simulink model "exp5"  (R2024b)
settings: Solver=ode4  StartTime=0.0  StopTime=.1  FixedStep=1e-8  RelTol=1e-3
libraries: spsDiodeLib x8, spsThyristorLib x8, spsSeriesRLCBranchLib x6, spsACVoltageSourceLib x4, spsCurrentMeasurementLib x4, spsMultimeterLib x4, spsMonostableLib x2, simulink x1, sps_lib x1
settings Model: Creator=91798  LastModifiedBy=91798
settings RTWCC: GPUComputeCapability=3.5

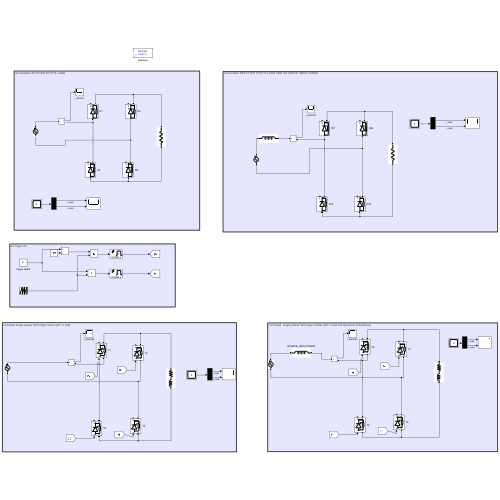
[thumbnail: Simulink's stored preview of the top-level diagram]
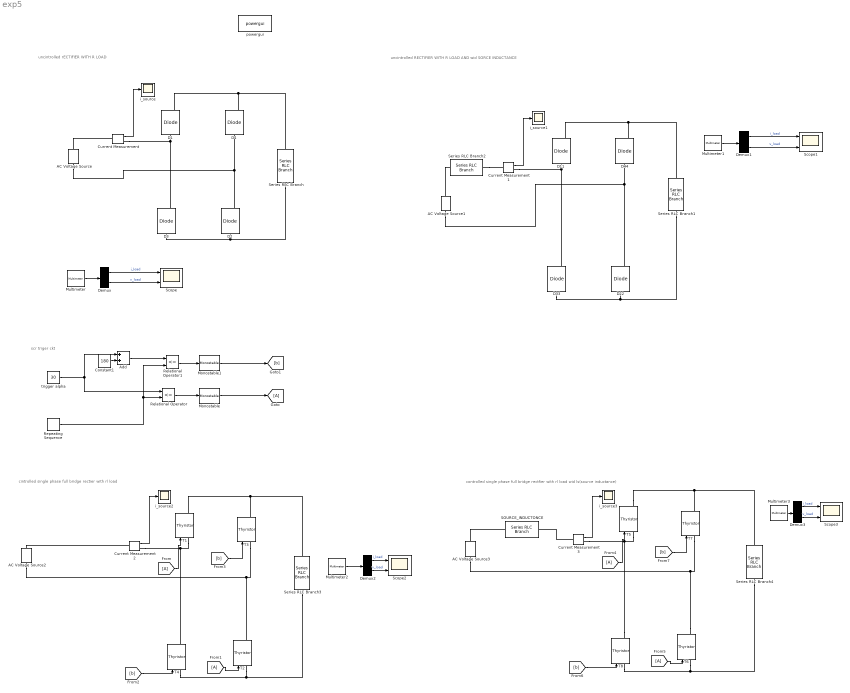
== system exp5 ==
  note: cintrolled single phase full bridge rectier with rl load
  note: controlled single phase full bridge rectfier with rl load wid ls(source inductance)
  note: scr triger ckt
  note: uncintrolled rECTIFIER WITH R LOAD
  note: uncintrolled RECTIFIER WITH R LOAD AND wid SORCE INDUCTANCE
  AC Voltage Source{,1..3} (4 alike) : spsACVoltageSourceLib/AC Voltage Source  Amplitude=230*sqrt(2)  Phase=0  Frequency=50  SampleTime=0  Measurements=None  BusType=swing  Pref=10e3  Qref=0  Qmin=-inf  Qmax=+inf
  Add : Sum
  Constant1 : Constant  Value=180
  Current Measurement{,1..3} (4 alike) : spsCurrentMeasurementLib/Current Measurement  PhasorSimulation=off  OutputType=Complex  PSBequivalent=0
  D{1..4} (4 alike) : spsDiodeLib/Diode  Ron=0.001  Lon=0  Vf=0.8  IC=0  UseSnubber=0  Rs=500  Cs=250e-9  Measurements=on
  D{11,22,33,44} (4 alike) : spsDiodeLib/Diode  Ron=0.001  Lon=0  Vf=0.8  IC=0  UseSnubber=0  Rs=5e10  Cs=inf  Measurements=on
  Demux{,1..3} (4 alike) : Demux  Outputs=2
  From{,1,4..5} (4 alike) : From
  Goto : Goto
  Monostable : spsMonostableLib/Monostable  EdgeDetect=Rising  PulseDuration=0.5e-3  ic=0  Ts=0
      settings: LibrarySourceBlock=sps_lib/Control/Monostable
  Monostable1 : spsMonostableLib/Monostable  EdgeDetect=Rising  PulseDuration=0.5e-3  ic=0  Ts=0
      settings: LibrarySourceBlock=sps_lib/Control/Monostable
  Multimeter : spsMultimeterLib/Multimeter  L=10  sel=[6 1]  yselected={}  Gain=[1 1]  OutputType=Complex  PlotAtSimulationStop=off  PhasorSimulation=off
  Multimeter1 : spsMultimeterLib/Multimeter  L=10  sel=[7 2]  yselected={}  Gain=[1 1]  OutputType=Complex  PlotAtSimulationStop=off  PhasorSimulation=off
  Multimeter2 : spsMultimeterLib/Multimeter  L=10  sel=[9 4]  yselected={}  Gain=[1 1]  OutputType=Complex  PlotAtSimulationStop=off  PhasorSimulation=off
  Multimeter3 : spsMultimeterLib/Multimeter  L=10  sel=[10 5]  yselected={}  Gain=[1 1]  OutputType=Complex  PlotAtSimulationStop=off  PhasorSimulation=off
  Relational Operator : RelationalOperator  Operator=<=  OutDataTypeStr=boolean  InputSameDT=off
  Relational Operator1 : RelationalOperator  Operator=<=  OutDataTypeStr=boolean  InputSameDT=off
  Repeating Sequence : simulink/Sources/Repeating Sequence  rep_seq_t=[0 .02]  rep_seq_y=[0 360]
  SOURCE_INDUCTONCE : spsSeriesRLCBranchLib/Series RLC Branch  LConnTagsString=__new0  RConnTagsString=__new0  BranchType=L  Resistance=20  Inductance=10e-3  SetiL0=off  InitialCurrent=0  Capacitance=1e-6  Setx0=off  InitialVoltage=0  Measurements=None
  Scope{,1..3} (4 alike) : Scope  NumInputPorts=2
  Series RLC Branch : spsSeriesRLCBranchLib/Series RLC Branch  LConnTagsString=__new0  RConnTagsString=__new0  BranchType=R  Resistance=20  Inductance=1e-3  SetiL0=off  InitialCurrent=0  Capacitance=1e-6  Setx0=off  InitialVoltage=0  Measurements=Branch voltage and current
  Series RLC Branch1 : spsSeriesRLCBranchLib/Series RLC Branch  LConnTagsString=__new0  RConnTagsString=__new0  BranchType=R  Resistance=20  Inductance=1e-3  SetiL0=off  InitialCurrent=0  Capacitance=1e-6  Setx0=off  InitialVoltage=0  Measurements=Branch voltage and current
  Series RLC Branch2 : spsSeriesRLCBranchLib/Series RLC Branch  LConnTagsString=__new0  RConnTagsString=__new0  BranchType=L  Resistance=20  Inductance=10e-3  SetiL0=off  InitialCurrent=0  Capacitance=1e-6  Setx0=off  InitialVoltage=0  Measurements=Branch voltage and current
  Series RLC Branch3 : spsSeriesRLCBranchLib/Series RLC Branch  LConnTagsString=__new0  RConnTagsString=__new0  BranchType=RL  Resistance=20  Inductance=200e-3  SetiL0=off  InitialCurrent=0  Capacitance=1e-6  Setx0=off  InitialVoltage=0  Measurements=Branch voltage and current
  Series RLC Branch4 : spsSeriesRLCBranchLib/Series RLC Branch  LConnTagsString=__new0  RConnTagsString=__new0  BranchType=RL  Resistance=20  Inductance=200e-3  SetiL0=off  InitialCurrent=0  Capacitance=1e-6  Setx0=off  InitialVoltage=0  Measurements=Branch voltage and current
  T{1..8} (8 alike) : spsThyristorLib/Thyristor  Ron=0.001  Lon=0  Vf=0.8  IC=0  Rs=500  Cs=250e-9  Measurements=on
  i_source{,1..3} (4 alike) : Scope
  powergui : sps_lib/powergui  Priority=1  SimulationMode=Discrete  SampleTime=5e-7  frequency=60  Iterations=50  frequencyindice=50  Pbase=100e6  ErrMax=1e-4  UnitsV=kV  UnitsW=MW  buscounter=0  FunctionMessages=off  echomessages=off  EnableUseOfTLC=off  CurrentSourceSwitches=off  DisableSnubberDevices=off  DisableRonSwitches=off  DisableVfSwitches=off  DisplayEquations=off  AutomaticDiscreteSolvers=off  SolverType=Tustin/Backward Euler (TBE)  Interpol=off  ExternalGateDelay=off  methode=off  Ts=100  x0status=blocks  SPID=on  SwTol=0  HookPort=off  NonlinearTolerance=1e-4  nMaxIteration=100  ContinueOnMaxIteration=off  RestoreLinks=warning  ResistiveCurrentMeasurement=off  Frange=[0:2:500]  Ylog=off  Xlog=on  ShowGrid=off  save=off  variable=ZData  structure=0  ZoomFFT=off  StartTime=0.0  cycles=1  DisplayStyle=1  fundamental=60  FreqAxis=off  MaxFrequency=1000  frequencyindicesteady=1  RmsSteady=1  display=off
  trigger alpha : Constant  Value=30
  wires:
  Current Measurement/1 -> i_source/1
  Demux/2 -> Scope/2  "v_load"
  Multimeter/1 -> Demux/1
  Demux/1 -> Scope/1  "i_load"
  Demux1/1 -> Scope1/1  "i_load"
  Multimeter1/1 -> Demux1/1
  Demux1/2 -> Scope1/2  "v_load"
  Current Measurement1/1 -> i_source1/1
  Multimeter2/1 -> Demux2/1
  Demux2/1 -> Scope2/1  "i_load"
  Demux2/2 -> Scope2/2  "v_load"
  Current Measurement2/1 -> i_source2/1
  trigger alpha/1 -> Add/1, Relational Operator/1
  Repeating Sequence/1 -> Relational Operator/2, Relational Operator1/2
  Relational Operator/1 -> Monostable/1
  Monostable/1 -> Goto/1
  Constant1/1 -> Add/2
  Add/1 -> Relational Operator1/1
  Relational Operator1/1 -> Monostable1/1
  Monostable1/1 -> [b]
  From/1 -> T1/1
  From1/1 -> T2/1
  [b] -> T4/1
  [b] -> T3/1
  From5/1 -> T6/1
  [b] -> T7/1
  From4/1 -> T5/1
  [b] -> T8/1
  Current Measurement3/1 -> i_source3/1
  Demux3/1 -> Scope3/1  "i_load"
  Multimeter3/1 -> Demux3/1
  Demux3/2 -> Scope3/2  "v_load"
  connections:
  D1/RConn1 -- Series RLC Branch/LConn1 -- D4/RConn1
  D3/RConn1 -- Current Measurement/RConn1 -- D1/LConn1
  D2/RConn1 -- AC Voltage Source/LConn1 -- D4/LConn1
  D3/LConn1 -- Series RLC Branch/RConn1 -- D2/LConn1
  AC Voltage Source/RConn1 -- Current Measurement/LConn1
  D11/LConn1 -- D33/RConn1 -- Current Measurement1/RConn1
  D11/RConn1 -- Series RLC Branch1/LConn1 -- D44/RConn1
  D22/RConn1 -- AC Voltage Source1/LConn1 -- D44/LConn1
  D22/LConn1 -- D33/LConn1 -- Series RLC Branch1/RConn1
  Series RLC Branch2/LConn1 -- Current Measurement1/LConn1
  AC Voltage Source1/RConn1 -- Series RLC Branch2/RConn1
  Series RLC Branch3/LConn1 -- T3/RConn1 -- T1/RConn1
  Series RLC Branch3/RConn1 -- T2/LConn1 -- T4/LConn1
  AC Voltage Source2/LConn1 -- T3/LConn1 -- T2/RConn1
  Current Measurement2/RConn1 -- T1/LConn1 -- T4/RConn1
  Current Measurement2/LConn1 -- AC Voltage Source2/RConn1
  T5/RConn1 -- Series RLC Branch4/LConn1 -- T7/RConn1
  T8/RConn1 -- Current Measurement3/RConn1 -- T5/LConn1
  T8/LConn1 -- Series RLC Branch4/RConn1 -- T6/LConn1
  T6/RConn1 -- AC Voltage Source3/LConn1 -- T7/LConn1
  SOURCE_INDUCTONCE/RConn1 -- AC Voltage Source3/RConn1
  Current Measurement3/LConn1 -- SOURCE_INDUCTONCE/LConn1
